simulink model "Discrete_sim_3R_scalar"  (R2024b)
settings: Solver=FixedStepAuto  StartTime=0.0  StopTime=22  FixedStep=0.1  MaxStep=0.1  RelTol=1e-3
libraries: simulink x1
(part 1 of 2)
settings Model: Creator=RSL  LastModifiedBy=cwaight
settings SolverCC: AlgebraicLoopSolver=TrustRegion
settings DataIOCC: ReturnWorkspaceOutputs=off
settings DebuggingCC: UnconnectedInputMsg=warning  UnconnectedOutputMsg=warning  UnconnectedLineMsg=warning  UnderSpecifiedDimensionMsg=warning  ArithmeticOperatorsInVariantConditions=warning
settings ModelReferenceCC: EnableRefExpFcnMdlSchedulingChecks=on
settings SFSimCC: SimUseLocalCustomCode=off  CustomCodeUndefinedFunction=UseInterfaceOnly
settings RTWCC: RTWUseLocalCustomCode=off  GPUComputeCapability=3.5
settings CodeAppCC: StateflowObjectComments=on

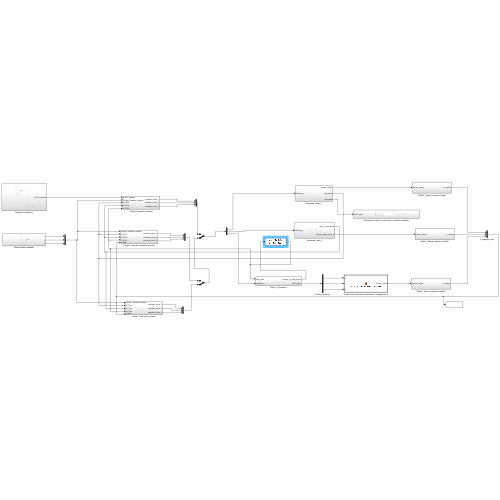
[thumbnail: Simulink's stored preview of the top-level diagram]
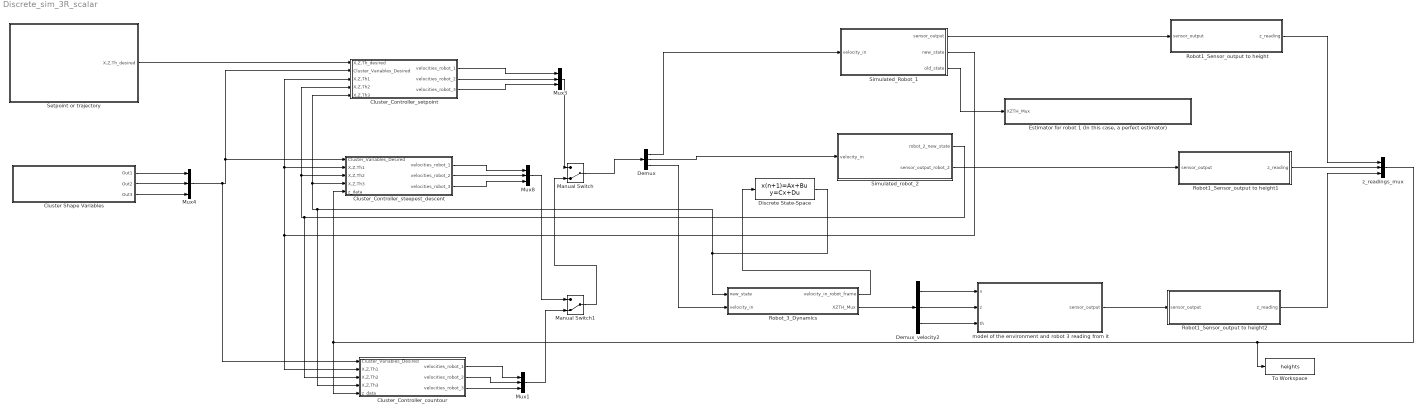
== system Discrete_sim_3R_scalar ==
  Cluster Shape Variables : Subsystem
  Cluster_Controller_countour : Subsystem
  Cluster_Controller_setpoint : Subsystem
  Cluster_Controller_steepest_descent : Subsystem
  Demux : Demux  Outputs=3
  Demux_velocity2 : Demux  Outputs=3
  Discrete State-Space : DiscreteStateSpace  A=[1 0 0; 0 1 0; 0 0 1]  B=[0.1 0 0; 0 0.10 0; 0 0 0.1]  C=[1 0 0; 0 1 0; 0 0 1]  D=[0 0 0; 0 0 0; 0 0 0]  InitialCondition=[-0.85,-1.1,0.1]  SampleTime=-1
  "Estimator for robot 1 (In this case, a perfect estimator)" : Subsystem
  Manual Switch : ManualSwitch  CurrentSetting=0
  Manual Switch1 : ManualSwitch  CurrentSetting=0
  Mux{1,3..4,8} (4 alike) : Mux  Inputs=3
  Robot1_Sensor_output to height : Subsystem
  Robot1_Sensor_output to height1 : Subsystem
  Robot1_Sensor_output to height2 : Subsystem
  Robot_3_Dynamics : Subsystem
  Setpoint or trajectory : Subsystem
  Simulated_Robot_1 : Subsystem
  Simulated_robot_2 : Subsystem
  To Workspace : ToWorkspace  VariableName=heights  SaveFormat=Timeseries  SampleTime=-1
  model of the environment and robot 3 reading from it : MATLAB Function  TreatAsAtomicUnit=on
  z_readings_mux : Mux  Inputs=3
  wires:
  Cluster_Controller_setpoint/1(velocities_robot_1) -> Mux3/1
  Cluster_Controller_setpoint/3(velocities_robot_3) -> Mux3/3
  Cluster_Controller_setpoint/2(velocities_robot_2) -> Mux3/2
  Mux4/1 -> Cluster_Controller_countour/1(Cluster_Variables_Desired), Cluster_Controller_steepest_descent/1(Cluster_Variables_Desired), Cluster_Controller_setpoint/2(Cluster_Variables_Desired)
  Cluster Shape Variables/1(Out1) -> Mux4/1
  Cluster Shape Variables/3(Out3) -> Mux4/3
  Setpoint or trajectory/1(X,Z,Th_desired) -> Cluster_Controller_setpoint/1(X,Z,Th_desired)
  Robot1_Sensor_output to height/1(z_reading) -> z_readings_mux/1
  Cluster_Controller_steepest_descent/3(velocities_robot_3) -> Mux8/3
  Cluster_Controller_steepest_descent/2(velocities_robot_2) -> Mux8/2
  Cluster_Controller_steepest_descent/1(velocities_robot_1) -> Mux8/1
  Cluster Shape Variables/2(Out2) -> Mux4/2
  Demux_velocity2/1 -> model of the environment and robot 3 reading from it/1(x)
  model of the environment and robot 3 reading from it/1(sensor_output) -> Robot1_Sensor_output to height2/1(sensor_output)
  Demux_velocity2/2 -> model of the environment and robot 3 reading from it/2(z)
  Demux_velocity2/3 -> model of the environment and robot 3 reading from it/3(th)
  Robot1_Sensor_output to height1/1(z_reading) -> z_readings_mux/2
  Robot1_Sensor_output to height2/1(z_reading) -> z_readings_mux/3
  Robot_3_Dynamics/2(XZTH_Mux) -> Demux_velocity2/1
  z_readings_mux/1 -> Cluster_Controller_steepest_descent/5(z_data), Cluster_Controller_countour/5(z_data), To Workspace/1
  Robot_3_Dynamics/1(velocity_in_robot_frame) -> Discrete State-Space/1
  Discrete State-Space/1 -> Robot_3_Dynamics/1(new_state), Cluster_Controller_countour/4(X,Z,Th3), Cluster_Controller_steepest_descent/4(X,Z,Th3), Cluster_Controller_setpoint/5(X,Z,Th3)
  Mux3/1 -> Manual Switch/1
  Simulated_Robot_1/2(new_state) -> Cluster_Controller_setpoint/3(X,Z,Th1), Cluster_Controller_steepest_descent/2(X,Z,Th1), Cluster_Controller_countour/2(X,Z,Th1)
  Simulated_Robot_1/1(sensor_output) -> Robot1_Sensor_output to height/1(sensor_output)
  Simulated_Robot_1/3(old_state) -> "Estimator for robot 1 (In this case, a perfect estimator)"/1(XZTH_Mux)
  Demux/1 -> Simulated_Robot_1/1(velocity_in)
  Manual Switch/1 -> Demux/1
  Simulated_robot_2/1(robot_2_new_state) -> Cluster_Controller_countour/3(X,Z,Th2), Cluster_Controller_setpoint/4(X,Z,Th2), Cluster_Controller_steepest_descent/3(X,Z,Th2)
  Demux/2 -> Simulated_robot_2/1(velocity_in)
  Simulated_robot_2/2(sensor_output_robot_2) -> Robot1_Sensor_output to height1/1(sensor_output)
  Demux/3 -> Robot_3_Dynamics/2(velocity_in)
  Manual Switch1/1 -> Manual Switch/2
  Mux8/1 -> Manual Switch1/1
  Mux1/1 -> Manual Switch1/2
  Cluster_Controller_countour/1(velocities_robot_1) -> Mux1/1
  Cluster_Controller_countour/2(velocities_robot_2) -> Mux1/2
  Cluster_Controller_countour/3(velocities_robot_3) -> Mux1/3

== system Discrete_sim_3R_scalar/Cluster Shape Variables ==
  Cluster Variable C : Constant  Value=pi/2
  Cluster_Variable_B : Constant  Value=0.35
  Cluster_variable_A : Constant  Value=0.35
  Out1 : Outport
  Out2 : Outport  Port=2
  Out3 : Outport  Port=3
  wires:
  Cluster_variable_A/1 -> Out1/1
  Cluster Variable C/1 -> Out3/1
  Cluster_Variable_B/1 -> Out2/1

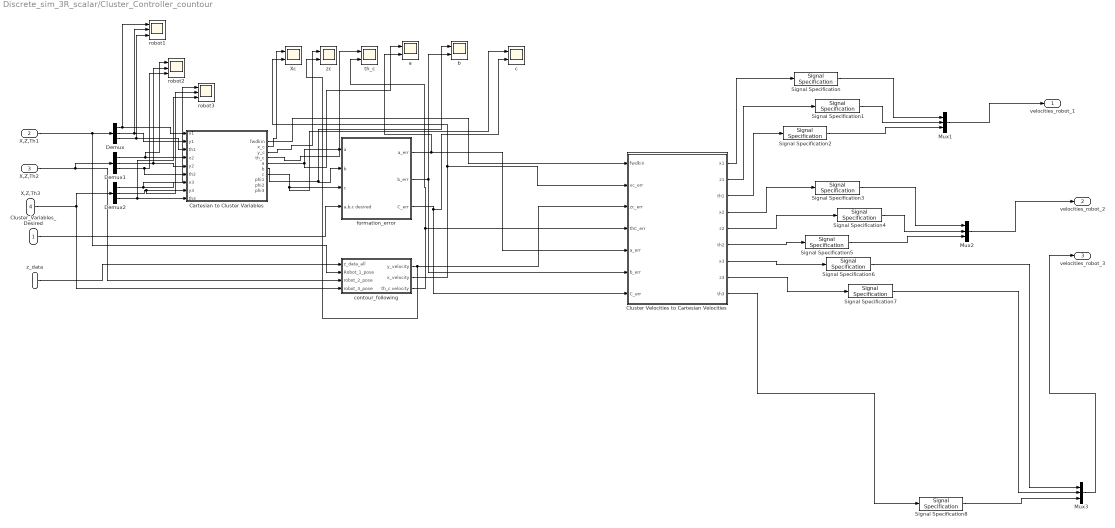
== system Discrete_sim_3R_scalar/Cluster_Controller_countour ==
  Cluster_Variables_Desired : Inport
  X,Z,Th1 : Inport  Port=2
  X,Z,Th2 : Inport  Port=3
  X,Z,Th3 : Inport  Port=4
  z_data : Inport  Port=5
  Cartesian to Cluster Variables : MATLAB Function  TreatAsAtomicUnit=on
  Cluster Velocities to Cartesian Velocities : MATLAB Function  TreatAsAtomicUnit=on
  Demux : Demux  Outputs=3
  Demux1 : Demux  Outputs=3
  Demux2 : Demux  Outputs=3
  Mux1 : Mux  Inputs=3
  Mux2 : Mux  Inputs=3
  Mux3 : Mux  Inputs=3
  Signal Specification{,1..8} (9 alike) : SignalSpecification  Dimensions=1
  Xc : Scope  NumInputPorts=2
  a : Scope  NumInputPorts=2
  b : Scope  NumInputPorts=2
  c : Scope  NumInputPorts=2
  contour_following : Subsystem
  formation_error : Subsystem
  robot1 : Scope  NumInputPorts=3
  robot2 : Scope  NumInputPorts=3
  robot3 : Scope  NumInputPorts=3
  th_c : Scope  NumInputPorts=2
  zc : Scope  NumInputPorts=2
  velocities_robot_1 : Outport
  velocities_robot_2 : Outport  Port=2
  velocities_robot_3 : Outport  Port=3
  wires:
  X,Z,Th1/1 -> contour_following/2(Robot_1_pose), Demux/1
  X,Z,Th2/1 -> contour_following/3(robot_2_pose), Demux1/1
  X,Z,Th3/1 -> Demux2/1, contour_following/4(robot_3_pose)
  Demux/1 -> robot1/1, Cartesian to Cluster Variables/1(x1)
  Demux/2 -> robot1/2, Cartesian to Cluster Variables/2(y1)
  Demux/3 -> robot1/3, Cartesian to Cluster Variables/3(th1)
  Demux1/1 -> robot2/1, Cartesian to Cluster Variables/4(x2)
  Demux1/2 -> robot2/2, Cartesian to Cluster Variables/5(y2)
  Demux1/3 -> robot2/3, Cartesian to Cluster Variables/6(th2)
  Demux2/1 -> robot3/1, Cartesian to Cluster Variables/7(x3)
  Demux2/2 -> robot3/2, Cartesian to Cluster Variables/8(y3)
  Demux2/3 -> robot3/3, Cartesian to Cluster Variables/9(th3)
  Cartesian to Cluster Variables/2(x_c) -> Xc/1
  Cartesian to Cluster Variables/3(y_c) -> zc/1
  Cartesian to Cluster Variables/4(th_c) -> th_c/1
  Cartesian to Cluster Variables/5(a) -> a/1, formation_error/1(a)
  Cartesian to Cluster Variables/6(b) -> formation_error/2(b), b/1
  Cartesian to Cluster Variables/7(c) -> c/1, formation_error/3(c)
  Cluster_Variables_Desired/1 -> formation_error/4(a,b,c desired)
  formation_error/1(a_err) -> Cluster Velocities to Cartesian Velocities/5(a_err), a/2
  formation_error/2(b_err) -> Cluster Velocities to Cartesian Velocities/6(b_err), b/2
  formation_error/3(C_err) -> Cluster Velocities to Cartesian Velocities/7(C_err), c/2
  Cartesian to Cluster Variables/1(fwdkin) -> Cluster Velocities to Cartesian Velocities/1(fwdkin)
  z_data/1 -> contour_following/1(z_data_all)
  contour_following/2(x_velocity) -> Cluster Velocities to Cartesian Velocities/2(xc_err), Xc/2
  contour_following/1(y_velocity) -> Cluster Velocities to Cartesian Velocities/3(zc_err), zc/2
  contour_following/3(th_c velocity) -> th_c/2, Cluster Velocities to Cartesian Velocities/4(thC_err)
  Signal Specification/1 -> Mux1/1
  Cluster Velocities to Cartesian Velocities/1(x1) -> Signal Specification/1
  Cluster Velocities to Cartesian Velocities/5(z2) -> Signal Specification4/1
  Signal Specification7/1 -> Mux3/2
  Cluster Velocities to Cartesian Velocities/7(x3) -> Signal Specification6/1
  Cluster Velocities to Cartesian Velocities/6(th2) -> Signal Specification5/1
  Mux1/1 -> velocities_robot_1/1
  Cluster Velocities to Cartesian Velocities/4(x2) -> Signal Specification3/1
  Signal Specification1/1 -> Mux1/2
  Signal Specification8/1 -> Mux3/3
  Signal Specification6/1 -> Mux3/1
  Signal Specification3/1 -> Mux2/1
  Signal Specification5/1 -> Mux2/3
  Signal Specification2/1 -> Mux1/3
  Cluster Velocities to Cartesian Velocities/3(th1) -> Signal Specification2/1
  Mux3/1 -> velocities_robot_3/1
  Signal Specification4/1 -> Mux2/2
  Cluster Velocities to Cartesian Velocities/9(th3) -> Signal Specification8/1
  Cluster Velocities to Cartesian Velocities/2(z1) -> Signal Specification1/1
  Mux2/1 -> velocities_robot_2/1
  Cluster Velocities to Cartesian Velocities/8(z3) -> Signal Specification7/1

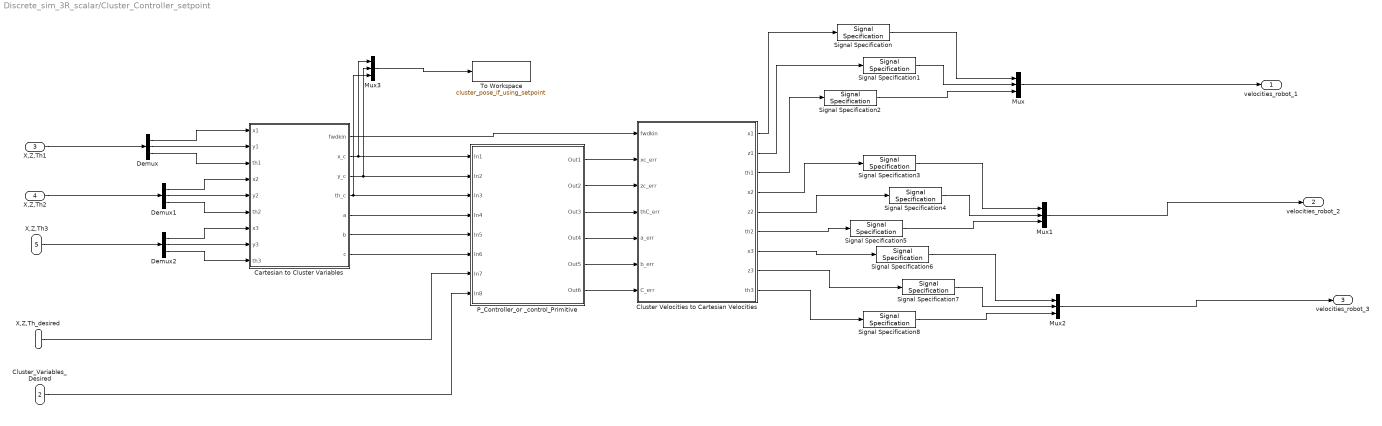
== system Discrete_sim_3R_scalar/Cluster_Controller_setpoint ==
  X,Z,Th_desired : Inport
  Cluster_Variables_Desired : Inport  Port=2
  X,Z,Th1 : Inport  Port=3
  X,Z,Th2 : Inport  Port=4
  X,Z,Th3 : Inport  Port=5
  Cartesian to Cluster Variables : MATLAB Function  TreatAsAtomicUnit=on
  Cluster Velocities to Cartesian Velocities : MATLAB Function  TreatAsAtomicUnit=on
  Demux : Demux  Outputs=3
  Demux1 : Demux  Outputs=3
  Demux2 : Demux  Outputs=3
  Mux{,1..3} (4 alike) : Mux  Inputs=3
  P_Controller_or _control_Primitive : Subsystem
  Signal Specification{,1..8} (9 alike) : SignalSpecification  Dimensions=1
  To Workspace : ToWorkspace  VariableName=cluster_pose_if_using_setpoint  SampleTime=-1
  velocities_robot_1 : Outport
  velocities_robot_2 : Outport  Port=2
  velocities_robot_3 : Outport  Port=3
  wires:
  X,Z,Th1/1 -> Demux/1
  X,Z,Th2/1 -> Demux1/1
  X,Z,Th3/1 -> Demux2/1
  Demux/1 -> Cartesian to Cluster Variables/1(x1)
  Demux/2 -> Cartesian to Cluster Variables/2(y1)
  Demux/3 -> Cartesian to Cluster Variables/3(th1)
  Demux1/1 -> Cartesian to Cluster Variables/4(x2)
  Demux1/2 -> Cartesian to Cluster Variables/5(y2)
  Demux1/3 -> Cartesian to Cluster Variables/6(th2)
  Demux2/1 -> Cartesian to Cluster Variables/7(x3)
  Demux2/2 -> Cartesian to Cluster Variables/8(y3)
  Demux2/3 -> Cartesian to Cluster Variables/9(th3)
  Cartesian to Cluster Variables/2(x_c) -> Mux3/1, P_Controller_or _control_Primitive/1(In1)
  Cartesian to Cluster Variables/3(y_c) -> Mux3/2, P_Controller_or _control_Primitive/2(In2)
  Cartesian to Cluster Variables/4(th_c) -> P_Controller_or _control_Primitive/3(In3), Mux3/3
  Cartesian to Cluster Variables/5(a) -> P_Controller_or _control_Primitive/4(In4)
  Cartesian to Cluster Variables/6(b) -> P_Controller_or _control_Primitive/5(In5)
  Cartesian to Cluster Variables/7(c) -> P_Controller_or _control_Primitive/6(In6)
  X,Z,Th_desired/1 -> P_Controller_or _control_Primitive/7(In7)
  Cluster_Variables_Desired/1 -> P_Controller_or _control_Primitive/8(In8)
  P_Controller_or _control_Primitive/1(Out1) -> Cluster Velocities to Cartesian Velocities/2(xc_err)
  P_Controller_or _control_Primitive/2(Out2) -> Cluster Velocities to Cartesian Velocities/3(zc_err)
  P_Controller_or _control_Primitive/3(Out3) -> Cluster Velocities to Cartesian Velocities/4(thC_err)
  P_Controller_or _control_Primitive/4(Out4) -> Cluster Velocities to Cartesian Velocities/5(a_err)
  P_Controller_or _control_Primitive/5(Out5) -> Cluster Velocities to Cartesian Velocities/6(b_err)
  P_Controller_or _control_Primitive/6(Out6) -> Cluster Velocities to Cartesian Velocities/7(C_err)
  Cartesian to Cluster Variables/1(fwdkin) -> Cluster Velocities to Cartesian Velocities/1(fwdkin)
  Mux/1 -> velocities_robot_1/1
  Signal Specification/1 -> Mux/1
  Cluster Velocities to Cartesian Velocities/1(x1) -> Signal Specification/1
  Signal Specification1/1 -> Mux/2
  Cluster Velocities to Cartesian Velocities/2(z1) -> Signal Specification1/1
  Signal Specification2/1 -> Mux/3
  Cluster Velocities to Cartesian Velocities/3(th1) -> Signal Specification2/1
  Signal Specification3/1 -> Mux1/1
  Cluster Velocities to Cartesian Velocities/4(x2) -> Signal Specification3/1
  Mux1/1 -> velocities_robot_2/1
  Signal Specification4/1 -> Mux1/2
  Signal Specification5/1 -> Mux1/3
  Cluster Velocities to Cartesian Velocities/6(th2) -> Signal Specification5/1
  Cluster Velocities to Cartesian Velocities/5(z2) -> Signal Specification4/1
  Signal Specification6/1 -> Mux2/1
  Cluster Velocities to Cartesian Velocities/7(x3) -> Signal Specification6/1
  Mux2/1 -> velocities_robot_3/1
  Signal Specification7/1 -> Mux2/2
  Signal Specification8/1 -> Mux2/3
  Cluster Velocities to Cartesian Velocities/9(th3) -> Signal Specification8/1
  Cluster Velocities to Cartesian Velocities/8(z3) -> Signal Specification7/1
  Mux3/1 -> To Workspace/1

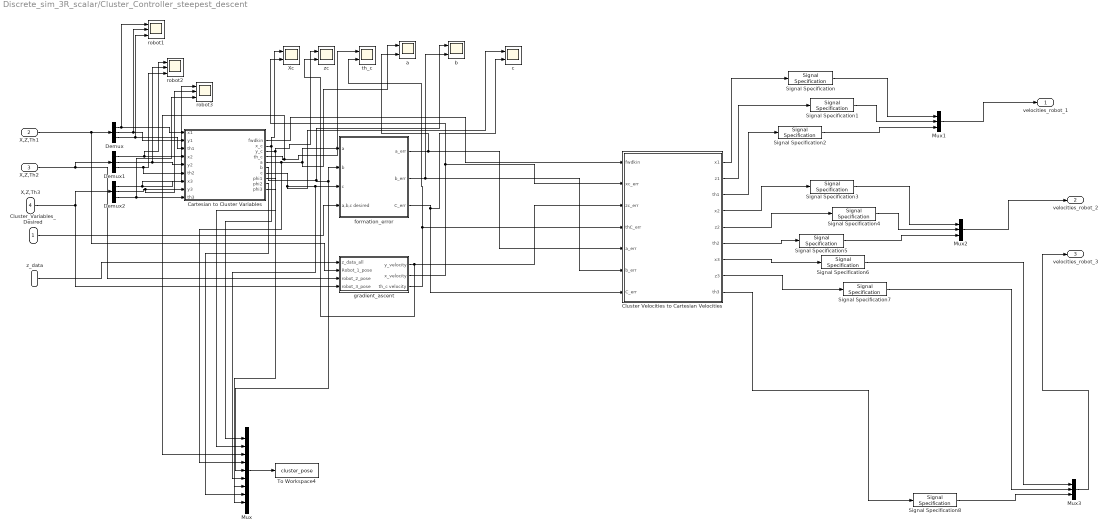
== system Discrete_sim_3R_scalar/Cluster_Controller_steepest_descent ==
  Cluster_Variables_Desired : Inport
  X,Z,Th1 : Inport  Port=2
  X,Z,Th2 : Inport  Port=3
  X,Z,Th3 : Inport  Port=4
  z_data : Inport  Port=5
  Cartesian to Cluster Variables : MATLAB Function  TreatAsAtomicUnit=on
  Cluster Velocities to Cartesian Velocities : MATLAB Function  TreatAsAtomicUnit=on
  Demux : Demux  Outputs=3
  Demux1 : Demux  Outputs=3
  Demux2 : Demux  Outputs=3
  Mux : Mux  Inputs=9
  Mux1 : Mux  Inputs=3
  Mux2 : Mux  Inputs=3
  Mux3 : Mux  Inputs=3
  Signal Specification{,1..8} (9 alike) : SignalSpecification  Dimensions=1
  To Workspace4 : ToWorkspace  VariableName=cluster_pose  SampleTime=-1
  Xc : Scope  NumInputPorts=2
  a : Scope  NumInputPorts=2
  b : Scope  NumInputPorts=2
  c : Scope  NumInputPorts=2
  formation_error : Subsystem
  gradient_ascent : Subsystem
  robot1 : Scope  NumInputPorts=3
  robot2 : Scope  NumInputPorts=3
  robot3 : Scope  NumInputPorts=3
  th_c : Scope  NumInputPorts=2
  zc : Scope  NumInputPorts=2
  velocities_robot_1 : Outport
  velocities_robot_2 : Outport  Port=2
  velocities_robot_3 : Outport  Port=3
  wires:
  X,Z,Th1/1 -> gradient_ascent/2(Robot_1_pose), Demux/1
  X,Z,Th2/1 -> gradient_ascent/3(robot_2_pose), Demux1/1
  X,Z,Th3/1 -> Demux2/1, gradient_ascent/4(robot_3_pose)
  Demux/1 -> robot1/1, Cartesian to Cluster Variables/1(x1)
  Demux/2 -> robot1/2, Cartesian to Cluster Variables/2(y1)
  Demux/3 -> robot1/3, Cartesian to Cluster Variables/3(th1)
  Demux1/1 -> robot2/1, Cartesian to Cluster Variables/4(x2)
  Demux1/2 -> robot2/2, Cartesian to Cluster Variables/5(y2)
  Demux1/3 -> robot2/3, Cartesian to Cluster Variables/6(th2)
  Demux2/1 -> robot3/1, Cartesian to Cluster Variables/7(x3)
  Demux2/2 -> robot3/2, Cartesian to Cluster Variables/8(y3)
  Demux2/3 -> robot3/3, Cartesian to Cluster Variables/9(th3)
  Cartesian to Cluster Variables/2(x_c) -> Xc/1, Mux/1
  Cartesian to Cluster Variables/3(y_c) -> zc/1, Mux/2
  Cartesian to Cluster Variables/4(th_c) -> Mux/3, th_c/1
  Cartesian to Cluster Variables/5(a) -> a/1, formation_error/1(a), Mux/4
  Cartesian to Cluster Variables/6(b) -> formation_error/2(b), Mux/5, b/1
  Cartesian to Cluster Variables/7(c) -> c/1, Mux/6, formation_error/3(c)
  Cluster_Variables_Desired/1 -> formation_error/4(a,b,c desired)
  formation_error/1(a_err) -> Cluster Velocities to Cartesian Velocities/5(a_err), a/2
  formation_error/2(b_err) -> Cluster Velocities to Cartesian Velocities/6(b_err), b/2
  formation_error/3(C_err) -> Cluster Velocities to Cartesian Velocities/7(C_err), c/2
  Cartesian to Cluster Variables/1(fwdkin) -> Cluster Velocities to Cartesian Velocities/1(fwdkin)
  z_data/1 -> gradient_ascent/1(z_data_all)
  gradient_ascent/2(x_velocity) -> Cluster Velocities to Cartesian Velocities/2(xc_err), Xc/2
  gradient_ascent/1(y_velocity) -> Cluster Velocities to Cartesian Velocities/3(zc_err), zc/2
  gradient_ascent/3(th_c velocity) -> th_c/2, Cluster Velocities to Cartesian Velocities/4(thC_err)
  Mux/1 -> To Workspace4/1
  Cartesian to Cluster Variables/8(phi1) -> Mux/7
  Cartesian to Cluster Variables/9(phi2) -> Mux/8
  Cartesian to Cluster Variables/10(phi3) -> Mux/9
  Signal Specification/1 -> Mux1/1
  Cluster Velocities to Cartesian Velocities/1(x1) -> Signal Specification/1
  Cluster Velocities to Cartesian Velocities/5(z2) -> Signal Specification4/1
  Signal Specification7/1 -> Mux3/2
  Cluster Velocities to Cartesian Velocities/7(x3) -> Signal Specification6/1
  Cluster Velocities to Cartesian Velocities/6(th2) -> Signal Specification5/1
  Mux1/1 -> velocities_robot_1/1
  Cluster Velocities to Cartesian Velocities/4(x2) -> Signal Specification3/1
  Signal Specification1/1 -> Mux1/2
  Signal Specification8/1 -> Mux3/3
  Signal Specification6/1 -> Mux3/1
  Signal Specification3/1 -> Mux2/1
  Signal Specification5/1 -> Mux2/3
  Signal Specification2/1 -> Mux1/3
  Cluster Velocities to Cartesian Velocities/3(th1) -> Signal Specification2/1
  Mux3/1 -> velocities_robot_3/1
  Signal Specification4/1 -> Mux2/2
  Cluster Velocities to Cartesian Velocities/9(th3) -> Signal Specification8/1
  Cluster Velocities to Cartesian Velocities/2(z1) -> Signal Specification1/1
  Mux2/1 -> velocities_robot_2/1
  Cluster Velocities to Cartesian Velocities/8(z3) -> Signal Specification7/1

== system Discrete_sim_3R_scalar/Estimator for robot 1 (In this case, a perfect estimator) ==
  XZTH_Mux : Inport
  Demux_velocity2 : Demux  Outputs=3
  Same Crater Yet Again : MATLAB Function  TreatAsAtomicUnit=on
  To Workspace6 : ToWorkspace  VariableName=sensor1_estimate  SampleTime=-1
  wires:
  Same Crater Yet Again/1(sensor_output) -> To Workspace6/1
  Demux_velocity2/3 -> Same Crater Yet Again/3(th)
  XZTH_Mux/1 -> Demux_velocity2/1
  Demux_velocity2/2 -> Same Crater Yet Again/2(z)
  Demux_velocity2/1 -> Same Crater Yet Again/1(x)

== system Discrete_sim_3R_scalar/Robot1_Sensor_output to height ==
  sensor_output : Inport
  Mountain : MATLAB Function  TreatAsAtomicUnit=on
  z_reading : Outport
  wires:
  sensor_output/1 -> Mountain/1(sensor_output)
  Mountain/1(height) -> z_reading/1

== system Discrete_sim_3R_scalar/Robot1_Sensor_output to height1 ==
  sensor_output : Inport
  Mountain : MATLAB Function  TreatAsAtomicUnit=on
  z_reading : Outport
  wires:
  sensor_output/1 -> Mountain/1(sensor_output)
  Mountain/1(height) -> z_reading/1

== system Discrete_sim_3R_scalar/Robot1_Sensor_output to height2 ==
  sensor_output : Inport
  Mountain : MATLAB Function  TreatAsAtomicUnit=on
  z_reading : Outport
  wires:
  sensor_output/1 -> Mountain/1(sensor_output)
  Mountain/1(height) -> z_reading/1

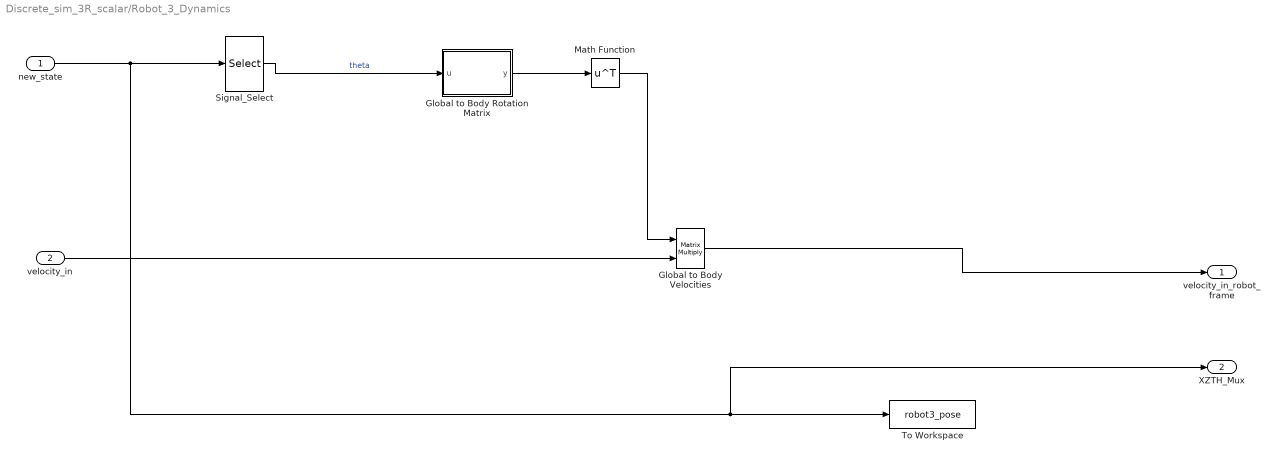
== system Discrete_sim_3R_scalar/Robot_3_Dynamics ==
  new_state : Inport
  velocity_in : Inport  Port=2
  Global to Body Velocities : Product  Multiplication=Matrix(*)
  Global to Body Rotation Matrix : MATLAB Function  TreatAsAtomicUnit=on
  Math Function : Math  Operator=transpose  SignedPower=on
  Signal_Select : Selector  InputPortWidth=3  IndexOptions=Index vector (dialog)  Indices=[3]  OutputSizes=1
  To Workspace : ToWorkspace  VariableName=robot3_pose  SaveFormat=Timeseries  SampleTime=-1
  velocity_in_robot_frame : Outport
  XZTH_Mux : Outport  Port=2
  wires:
  Signal_Select/1 -> Global to Body Rotation Matrix/1(u)  "theta"
  Global to Body Velocities/1 -> velocity_in_robot_frame/1
  new_state/1 -> XZTH_Mux/1, To Workspace/1, Signal_Select/1
  velocity_in/1 -> Global to Body Velocities/2
  Global to Body Rotation Matrix/1(y) -> Math Function/1
  Math Function/1 -> Global to Body Velocities/1

== system Discrete_sim_3R_scalar/Setpoint or trajectory ==
  Manual Switch : ManualSwitch
  Mux3 : Mux  Inputs=3
  Ramp : simulink/Sources/Ramp  slope=1  start=0  InitialOutput=0.1
  "Theta_Set Point1 " : Constant  Value=0.1
  X_Set Point : Constant  Value=1.5
  Z_Set Point1 : Constant  Value=0.5
  X,Z,Th_desired : Outport
  wires:
  Mux3/1 -> X,Z,Th_desired/1
  Z_Set Point1/1 -> Mux3/2
  Manual Switch/1 -> Mux3/3
  "Theta_Set Point1 "/1 -> Manual Switch/1
  X_Set Point/1 -> Mux3/1
  Ramp/1 -> Manual Switch/2

== system Discrete_sim_3R_scalar/Simulated_Robot_1 ==
  velocity_in : Inport
  Crater : MATLAB Function  TreatAsAtomicUnit=on
  Demux_velocity : Demux  Outputs=3
  Discrete State-Space : DiscreteStateSpace  A=[1 0 0; 0 1 0; 0 0 1]  B=[0.1 0 0; 0 0.10 0; 0 0 0.1]  C=[1 0 0; 0 1 0; 0 0 1]  D=[0 0 0; 0 0 0; 0 0 0]  InitialCondition=[-1,-1,0]  SampleTime=-1
  Robot_signal_processing_1 : Subsystem
  sensor_output : Outport
  new_state : Outport  Port=2
  old_state : Outport  Port=3
  wires:
  Crater/1(sensor_output) -> sensor_output/1
  Demux_velocity/1 -> Crater/1(x)
  Demux_velocity/3 -> Crater/3(th)
  Robot_signal_processing_1/2(XZTH_Mux) -> old_state/1, Demux_velocity/1
  velocity_in/1 -> Robot_signal_processing_1/2(velocity_in)
  Discrete State-Space/1 -> Robot_signal_processing_1/1(robot_1_pose), new_state/1
  Demux_velocity/2 -> Crater/2(z)
  Robot_signal_processing_1/1(velocity_in_robot_frame) -> Discrete State-Space/1

== system Discrete_sim_3R_scalar/Simulated_robot_2 ==
  velocity_in : Inport
  Demux_velocity1 : Demux  Outputs=3
  Discrete State-Space : DiscreteStateSpace  A=[1 0 0; 0 1 0; 0 0 1]  B=[0.1 0 0; 0 0.10 0; 0 0 0.1]  C=[1 0 0; 0 1 0; 0 0 1]  D=[0 0 0; 0 0 0; 0 0 0]  InitialCondition=[-1.1,-1.1,0]  SampleTime=-1
  Robot_signal_processing_2 : Subsystem
  Same Crater : MATLAB Function  TreatAsAtomicUnit=on
  robot_2_new_state : Outport
  sensor_output_robot_2 : Outport  Port=2
  wires:
  Demux_velocity1/1 -> Same Crater/1(x)
  Demux_velocity1/3 -> Same Crater/3(th)
  Same Crater/1(sensor_output) -> sensor_output_robot_2/1
  Demux_velocity1/2 -> Same Crater/2(z)
  velocity_in/1 -> Robot_signal_processing_2/2(velocity_in)
  Discrete State-Space/1 -> robot_2_new_state/1, Robot_signal_processing_2/1(robot_2)
  Robot_signal_processing_2/2(XZTH_Mux) -> Demux_velocity1/1
  Robot_signal_processing_2/1(velocity_in_robot_frame) -> Discrete State-Space/1

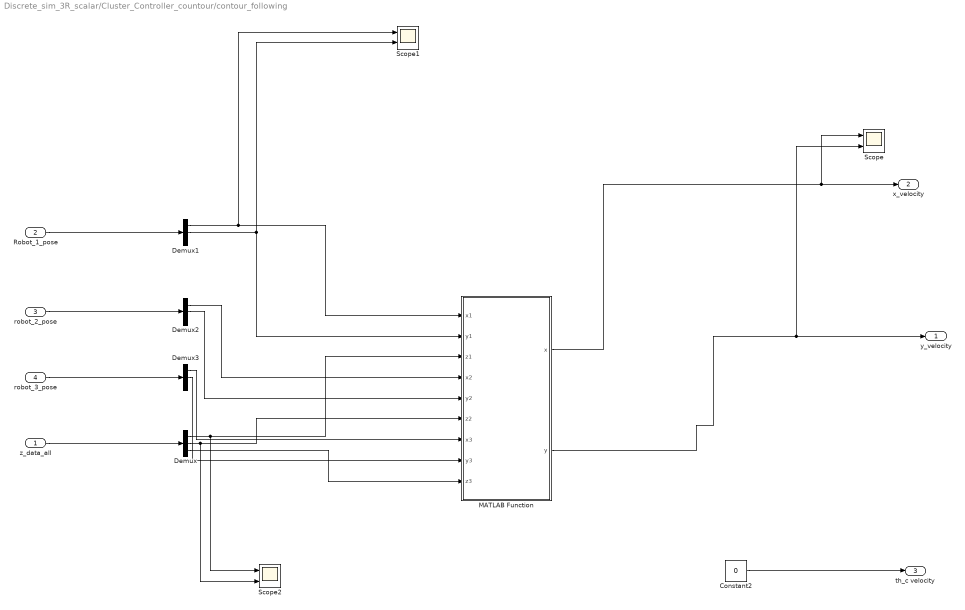
== system Discrete_sim_3R_scalar/Cluster_Controller_countour/contour_following ==
  z_data_all : Inport
  Robot_1_pose : Inport  Port=2
  robot_2_pose : Inport  Port=3
  robot_3_pose : Inport  Port=4
  Constant2 : Constant  Value=0
  Demux{,1..3} (4 alike) : Demux  Outputs=3
  MATLAB Function : MATLAB Function  TreatAsAtomicUnit=on
  Scope : Scope  NumInputPorts=2
  Scope1 : Scope  NumInputPorts=2
  Scope2 : Scope  NumInputPorts=2
  y_velocity : Outport
  x_velocity : Outport  Port=2
  th_c velocity : Outport  Port=3
  wires:
  Constant2/1 -> th_c velocity/1
  z_data_all/1 -> Demux/1
  Robot_1_pose/1 -> Demux1/1
  robot_2_pose/1 -> Demux2/1
  robot_3_pose/1 -> Demux3/1
  Demux1/1 -> Scope1/1, MATLAB Function/1(x1)
  Demux1/2 -> MATLAB Function/2(y1), Scope1/2
  Demux/1 -> Scope2/1, MATLAB Function/3(z1)
  Demux2/1 -> MATLAB Function/4(x2)
  Demux2/2 -> MATLAB Function/5(y2)
  Demux/2 -> Scope2/2, MATLAB Function/6(z2)
  Demux3/1 -> MATLAB Function/7(x3)
  Demux3/2 -> MATLAB Function/8(y3)
  Demux/3 -> MATLAB Function/9(z3)
  MATLAB Function/1(x) -> Scope/1, x_velocity/1
  MATLAB Function/2(y) -> Scope/2, y_velocity/1

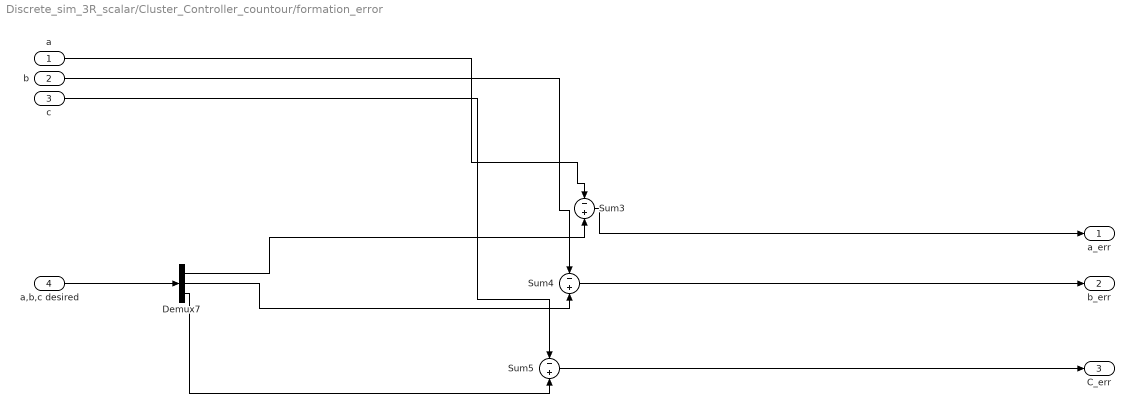
== system Discrete_sim_3R_scalar/Cluster_Controller_countour/formation_error ==
  a : Inport
  b : Inport  Port=2
  c : Inport  Port=3
  a,b,c desired : Inport  Port=4
  Demux7 : Demux  Outputs=3
  Sum3 : Sum  Inputs=-+
  Sum4 : Sum  Inputs=-+
  Sum5 : Sum  Inputs=-+
  a_err : Outport
  b_err : Outport  Port=2
  C_err : Outport  Port=3
  wires:
  Sum3/1 -> a_err/1
  Demux7/3 -> Sum5/2
  a,b,c desired/1 -> Demux7/1
  Demux7/1 -> Sum3/2
  b/1 -> Sum4/1
  Demux7/2 -> Sum4/2
  c/1 -> Sum5/1
  Sum4/1 -> b_err/1
  Sum5/1 -> C_err/1
  a/1 -> Sum3/1

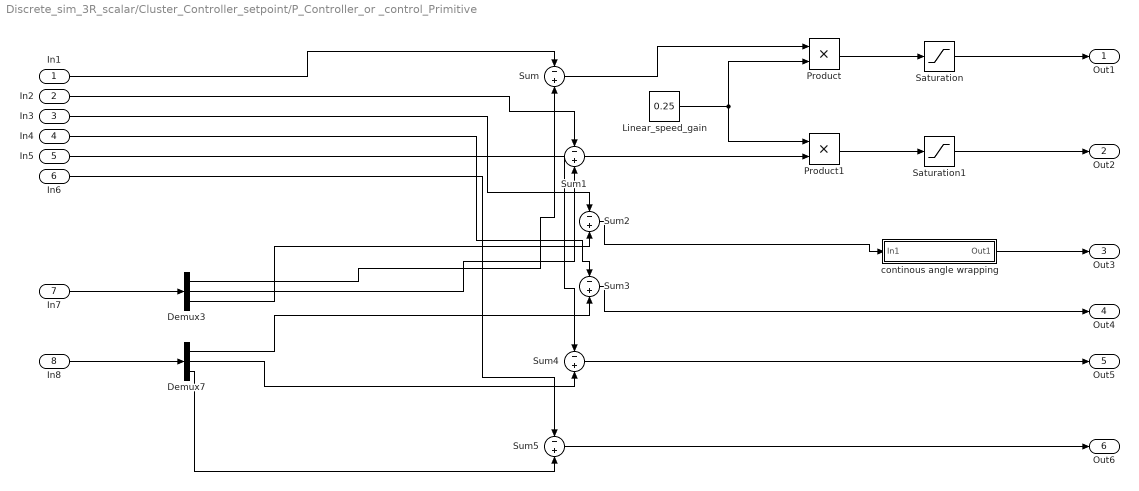
== system Discrete_sim_3R_scalar/Cluster_Controller_setpoint/P_Controller_or _control_Primitive ==
  In1 : Inport
  In2 : Inport  Port=2
  In3 : Inport  Port=3
  In4 : Inport  Port=4
  In5 : Inport  Port=5
  In6 : Inport  Port=6
  In7 : Inport  Port=7
  In8 : Inport  Port=8
  Demux3 : Demux  Outputs=3
  Demux7 : Demux  Outputs=3
  Linear_speed_gain : Constant  Value=0.25
  Product : Product
  Product1 : Product
  Saturation : Saturate
  Saturation1 : Saturate
  Sum{,1..5} (6 alike) : Sum  Inputs=-+
  continous angle wrapping : Subsystem
  Out1 : Outport
  Out2 : Outport  Port=2
  Out3 : Outport  Port=3
  Out4 : Outport  Port=4
  Out5 : Outport  Port=5
  Out6 : Outport  Port=6
  wires:
  In3/1 -> Sum2/1
  Demux3/2 -> Sum1/2
  Sum3/1 -> Out4/1
  In2/1 -> Sum1/1
  Demux3/3 -> Sum2/2
  Demux7/3 -> Sum5/2
  In8/1 -> Demux7/1
  Demux7/1 -> Sum3/2
  In1/1 -> Sum/1
  In5/1 -> Sum4/1
  Demux7/2 -> Sum4/2
  In6/1 -> Sum5/1
  Sum4/1 -> Out5/1
  Sum5/1 -> Out6/1
  Demux3/1 -> Sum/2
  In4/1 -> Sum3/1
  In7/1 -> Demux3/1
  Sum2/1 -> continous angle wrapping/1(In1)
  continous angle wrapping/1(Out1) -> Out3/1
  Sum/1 -> Product/1
  Linear_speed_gain/1 -> Product/2, Product1/1
  Sum1/1 -> Product1/2
  Saturation/1 -> Out1/1
  Product/1 -> Saturation/1
  Product1/1 -> Saturation1/1
  Saturation1/1 -> Out2/1

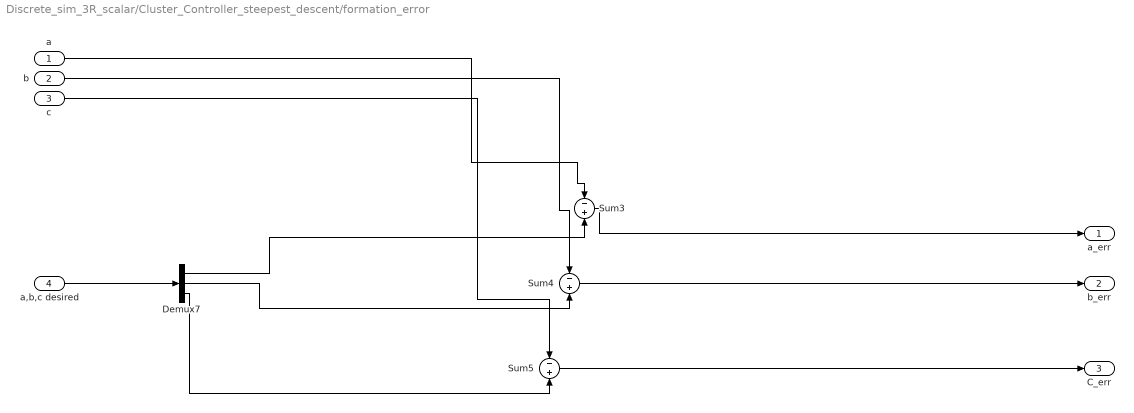
== system Discrete_sim_3R_scalar/Cluster_Controller_steepest_descent/formation_error ==
  a : Inport
  b : Inport  Port=2
  c : Inport  Port=3
  a,b,c desired : Inport  Port=4
  Demux7 : Demux  Outputs=3
  Sum3 : Sum  Inputs=-+
  Sum4 : Sum  Inputs=-+
  Sum5 : Sum  Inputs=-+
  a_err : Outport
  b_err : Outport  Port=2
  C_err : Outport  Port=3
  wires:
  Sum3/1 -> a_err/1
  Demux7/3 -> Sum5/2
  a,b,c desired/1 -> Demux7/1
  Demux7/1 -> Sum3/2
  b/1 -> Sum4/1
  Demux7/2 -> Sum4/2
  c/1 -> Sum5/1
  Sum4/1 -> b_err/1
  Sum5/1 -> C_err/1
  a/1 -> Sum3/1

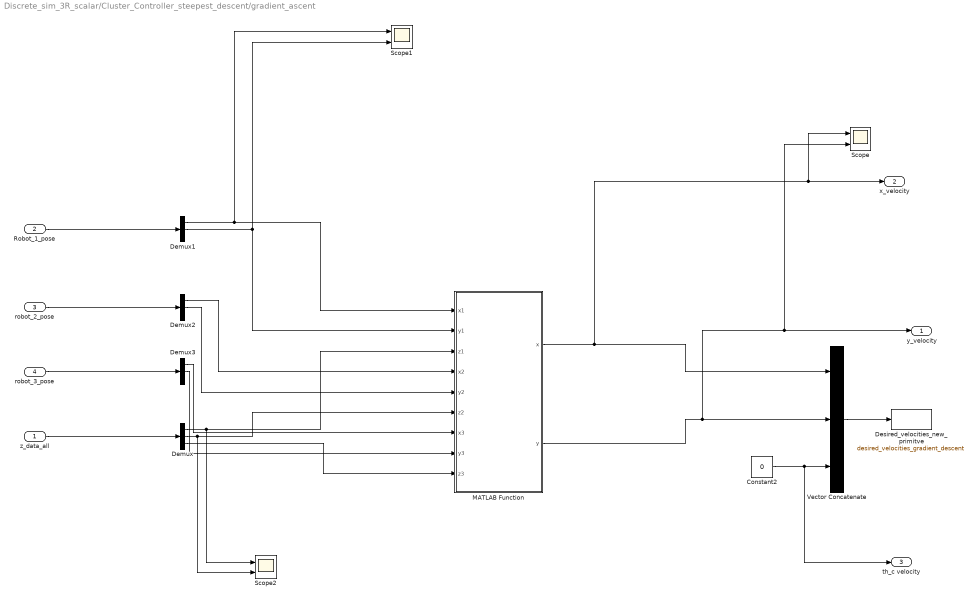
== system Discrete_sim_3R_scalar/Cluster_Controller_steepest_descent/gradient_ascent ==
  z_data_all : Inport
  Robot_1_pose : Inport  Port=2
  robot_2_pose : Inport  Port=3
  robot_3_pose : Inport  Port=4
  Constant2 : Constant  Value=0
  Demux{,1..3} (4 alike) : Demux  Outputs=3
  Desired_velocities_new_primitve : ToWorkspace  VariableName=desired_velocities_gradient_descent  SampleTime=-1
  MATLAB Function : MATLAB Function  TreatAsAtomicUnit=on
  Scope : Scope  NumInputPorts=2
  Scope1 : Scope  NumInputPorts=2
  Scope2 : Scope  NumInputPorts=2
  Vector Concatenate : Concatenate  NumInputs=3
  y_velocity : Outport
  x_velocity : Outport  Port=2
  th_c velocity : Outport  Port=3
  wires:
  Vector Concatenate/1 -> Desired_velocities_new_primitve/1
  Constant2/1 -> th_c velocity/1, Vector Concatenate/3
  z_data_all/1 -> Demux/1
  Robot_1_pose/1 -> Demux1/1
  robot_2_pose/1 -> Demux2/1
  robot_3_pose/1 -> Demux3/1
  Demux1/1 -> Scope1/1, MATLAB Function/1(x1)
  Demux1/2 -> MATLAB Function/2(y1), Scope1/2
  Demux/1 -> Scope2/1, MATLAB Function/3(z1)
  Demux2/1 -> MATLAB Function/4(x2)
  Demux2/2 -> MATLAB Function/5(y2)
  Demux/2 -> Scope2/2, MATLAB Function/6(z2)
  Demux3/1 -> MATLAB Function/7(x3)
  Demux3/2 -> MATLAB Function/8(y3)
  Demux/3 -> MATLAB Function/9(z3)
  MATLAB Function/1(x) -> Scope/1, x_velocity/1, Vector Concatenate/1
  MATLAB Function/2(y) -> Scope/2, y_velocity/1, Vector Concatenate/2

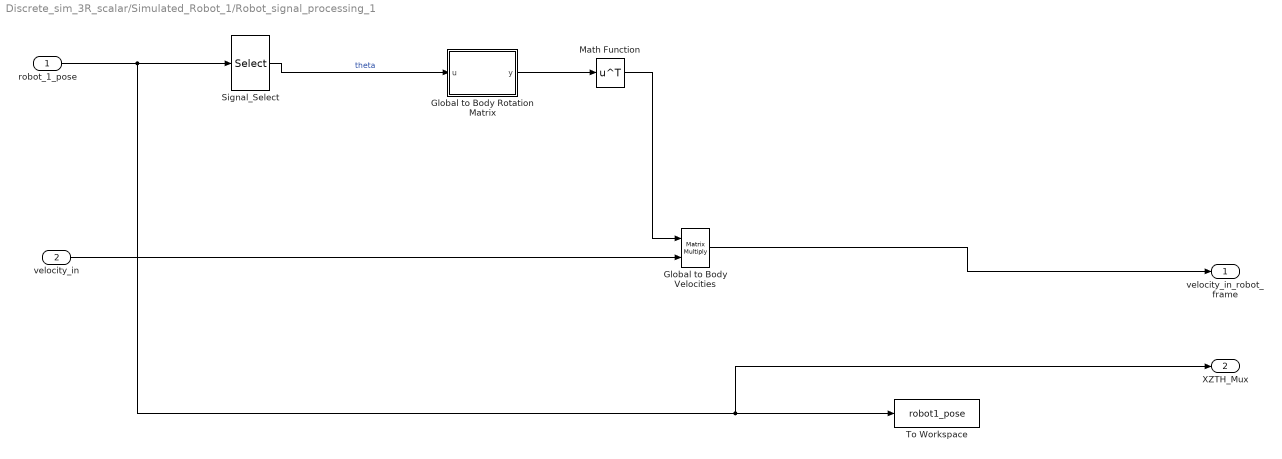
== system Discrete_sim_3R_scalar/Simulated_Robot_1/Robot_signal_processing_1 ==
  robot_1_pose : Inport
  velocity_in : Inport  Port=2
  Global to Body Velocities : Product  Multiplication=Matrix(*)
  Global to Body Rotation Matrix : MATLAB Function  TreatAsAtomicUnit=on
  Math Function : Math  Operator=transpose  SignedPower=on
  Signal_Select : Selector  InputPortWidth=3  IndexOptions=Index vector (dialog)  Indices=[3]  OutputSizes=1
  To Workspace : ToWorkspace  VariableName=robot1_pose  SaveFormat=Timeseries  SampleTime=-1
  velocity_in_robot_frame : Outport
  XZTH_Mux : Outport  Port=2
  wires:
  Signal_Select/1 -> Global to Body Rotation Matrix/1(u)  "theta"
  Global to Body Velocities/1 -> velocity_in_robot_frame/1
  robot_1_pose/1 -> XZTH_Mux/1, To Workspace/1, Signal_Select/1
  velocity_in/1 -> Global to Body Velocities/2
  Global to Body Rotation Matrix/1(y) -> Math Function/1
  Math Function/1 -> Global to Body Velocities/1

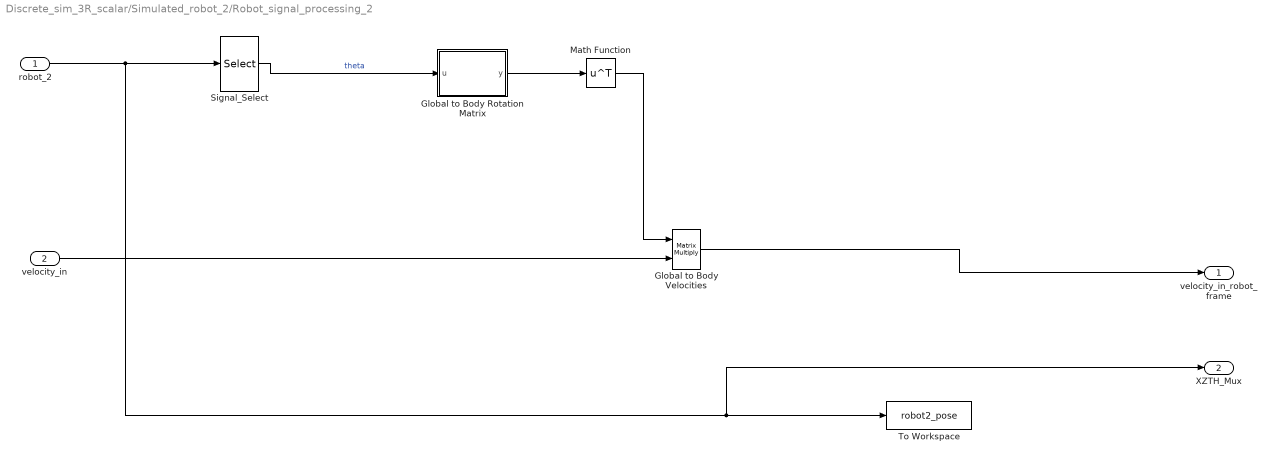
== system Discrete_sim_3R_scalar/Simulated_robot_2/Robot_signal_processing_2 ==
  robot_2 : Inport
  velocity_in : Inport  Port=2
  Global to Body Velocities : Product  Multiplication=Matrix(*)
  Global to Body Rotation Matrix : MATLAB Function  TreatAsAtomicUnit=on
  Math Function : Math  Operator=transpose  SignedPower=on
  Signal_Select : Selector  InputPortWidth=3  IndexOptions=Index vector (dialog)  Indices=[3]  OutputSizes=1
  To Workspace : ToWorkspace  VariableName=robot2_pose  SaveFormat=Timeseries  SampleTime=-1
  velocity_in_robot_frame : Outport
  XZTH_Mux : Outport  Port=2
  wires:
  Signal_Select/1 -> Global to Body Rotation Matrix/1(u)  "theta"
  Global to Body Velocities/1 -> velocity_in_robot_frame/1
  robot_2/1 -> XZTH_Mux/1, To Workspace/1, Signal_Select/1
  velocity_in/1 -> Global to Body Velocities/2
  Global to Body Rotation Matrix/1(y) -> Math Function/1
  Math Function/1 -> Global to Body Velocities/1

== system Discrete_sim_3R_scalar/Cluster_Controller_setpoint/P_Controller_or _control_Primitive/continous angle wrapping ==
  In1 : Inport
  Constant : Constant  Value=pi
  Constant1 : Constant  Value=2*pi
  Math Function : Math  Operator=mod  SignedPower=on
  Sum6 : Sum
  Sum7 : Sum  Inputs=-+
  Out1 : Outport
  wires:
  In1/1 -> Sum6/2
  Math Function/1 -> Sum7/2
  Constant/1 -> Sum7/1, Sum6/1
  Sum6/1 -> Math Function/1
  Constant1/1 -> Math Function/2
  Sum7/1 -> Out1/1

== matlab function Discrete_sim_3R_scalar/Cluster_Controller_countour/Cartesian to Cluster Variables ==
  data: fwdkin output; x1 input; x_c output; y1 input; th1 input; x2 input; y2 input; th2 input; x3 input; y3 input; th3 input; y_c output; th_c output; a output; b output; c output; phi1 output; phi2 output; phi3 output
function [fwdkin, x_c, y_c, th_c, a, b, c,phi1,phi2,phi3]   = Forward_Kinematics(x1, y1, th1, x2,y2,th2, x3,y3,th3)
% Centre frame
x_c = (x1+x2+x3)/3;
y_c = (y1+y2+y3)/3;
theta_c = atan2((2/3)*x1 - (1/3)*(x2 + x3), (2/3)*y1 - (1/3)*(y2 + y3));
% SAS Properties of triangle
p = sqrt((x1 - x2)^2 + (y1 - y2)^2);
q = sqrt((x3 - x1)^2 + (y1 - y3)^2);
beta = acos(((p^2 + q^2 - (x3 - x2)^2 - (y3 - y2)^2) / (2*p*q)));
% Rotation vectors
phi1 = th1 + theta_c;
phi2 = th2 + theta_c;
phi3 = th3 + theta_c;
a =p;
b = q;
c = beta;
th_c = theta_c;
fwdkin = [0 0 0 0 0 0];
fwdkin(1) =a;
fwdkin(2) =b;
fwdkin(3) =c;
fwdkin(4) =x_c;
fwdkin(5) =y_c;
fwdkin(6) =th_c;

== matlab function Discrete_sim_3R_scalar/Cluster_Controller_countour/Cluster Velocities to Cartesian Velocities ==
  data: fwdkin input; xc_err input; x1 output; zc_err input; thC_err input; a_err input; b_err input; C_err input; z1 output; th1 output; x2 output; z2 output; th2 output; x3 output; z3 output; th3 output
function [x1, z1,th1, x2,z2,th2, x3,z3, th3] = InverseJabobian(fwdkin, xc_err, zc_err, thC_err, a_err, b_err, C_err)
%% Unpacking the information from fwd_kin
p = fwdkin(1);
q = fwdkin(2);
beta = fwdkin(3);
xc = fwdkin(4);
yc = fwdkin(5);
theta_c = fwdkin(6);
yc_err = zc_err;
theta_c_err = thC_err;
p_err = a_err;
q_err = b_err;
beta_err = C_err;
%% Inverse Kinematics
  % Calculate x1, y1, and theta1 (Equations 12, 13, and 14)
r = sqrt((q + p*cos(beta))^2 + (p*sin(beta))^2);
  
x1 = xc + (1/3)*r*sin(theta_c);
y1 = yc + (1/3)*r*cos(theta_c);
%theta1 = phi1 - theta_c;
% Calculate x2, y2, and theta2 (Equations 15, 16, and 17)
x2 = xc + (1/3)*r*sin(theta_c) - p*sin(beta/2 + theta_c);
y2 = yc + (1/3)*r*cos(theta_c) - p*cos(beta/2 + theta_c);
%theta2 = phi2 - theta_c;
% Calculate x3, y3, and theta3 (Equations 18, 19, and 20)
x3 = xc + (1/3)*r*sin(theta_c) + q*sin(beta/2 - theta_c);
y3 = yc + (1/3)*r*cos(theta_c) - q*cos(beta/2 - theta_c);
%theta3 = phi3 - theta_c;
%% Now to take the partial derivates
% syms p q beta xc yc theta_c p_err q_err beta_err xc_err yc_err theta_c_err
% 
% % Define the equations
% eqs = [
%   xc + (1/3)*(sqrt((q + p*cos(beta))^2 + (p*sin(beta))^2))*sin(theta_c); % x1
%   yc + (1/3)*(sqrt((q + p*cos(beta))^2 + (p*sin(beta))^2))*cos(theta_c); % y1
%   xc + (1/3)*(sqrt((q + p*cos(beta))^2 + (p*sin(beta))^2))*sin(theta_c) - p*sin(beta/2 + theta_c); % x2
%   yc + (1/3)*(sqrt((q + p*cos(beta))^2 + (p*sin(beta))^2))*cos(theta_c) - p*cos(beta/2 + theta_c); % y2
%   xc + (1/3)*(sqrt((q + p*cos(beta))^2 + (p*sin(beta))^2))*sin(theta_c) + q*sin(beta/2 - theta_c); % x3
%   yc + (1/3)*(sqrt((q + p*cos(beta))^2 + (p*sin(beta))^2))*cos(theta_c) - q*cos(beta/2 - theta_c)  % y3
% ];
% 
% % Define the variables for differentiation
% vars = [p, q, beta, xc, yc, theta_c];
% 
% % Define the errors
% errs = [p_err, q_err, beta_err, xc_err, yc_err, theta_c_err];
% 
% % Initialize an array to store the sums (as symbolic)
% sums = sym(zeros(length(eqs), 1));
% 
% % Loop through equations and variables
% for i = 1:length(eqs)
%   for j = 1:length(vars)
%     derivative = diff(eqs(i), vars(j));
%     sums(i) = sums(i) + derivative * errs(j);
%   end
% end
% 
% % Display the results
% disp(simplify(sums(1)))
% disp(simplify(sums(2)))
% disp(simplify(sums(3)))
% disp(simplify(sums(4)))
% disp(simplify(sums(5)))
% disp(simplify(sums(6)))
%% Now to sum it all up
x1 =(3*xc_err*(p^2 + 2*cos(beta)*p*q + q^2)^(1/2) + p*p_err*sin(theta_c) + q*q_err*sin(theta_c) + p^2*theta_c_err*cos(theta_c) + q^2*theta_c_err*cos(theta_c) + p*q_err*cos(beta)*sin(theta_c) + p_err*q*cos(beta)*sin(theta_c) + 2*p*q*theta_c_err*cos(beta)*cos(theta_c) - beta_err*p*q*sin(beta)*sin(theta_c))/(3*(p^2 + 2*cos(beta)*p*q + q^2)^(1/2));
 
z1 = (3*yc_err*(p^2 + 2*cos(beta)*p*q + q^2)^(1/2) + p*p_err*cos(theta_c) + q*q_err*cos(theta_c) - p^2*theta_c_err*sin(theta_c) - q^2*theta_c_err*sin(theta_c) + p*q_err*cos(beta)*cos(theta_c) + p_err*q*cos(beta)*cos(theta_c) - beta_err*p*q*sin(beta)*cos(theta_c) - 2*p*q*theta_c_err*cos(beta)*sin(theta_c))/(3*(p^2 + 2*cos(beta)*p*q + q^2)^(1/2));
 
x2 = xc_err - p_err*(sin(beta/2 + theta_c) - (sin(theta_c)*(p + q*cos(beta)))/(3*(p^2 + 2*cos(beta)*p*q + q^2)^(1/2))) - beta_err*((p*cos(beta/2 + theta_c))/2 + (p*q*sin(beta)*sin(theta_c))/(3*(p^2 + 2*cos(beta)*p*q + q^2)^(1/2))) + theta_c_err*((cos(theta_c)*(p^2 + 2*cos(beta)*p*q + q^2)^(1/2))/3 - p*cos(beta/2 + theta_c)) + (q_err*sin(theta_c)*(q + p*cos(beta)))/(3*(p^2 + 2*cos(beta)*p*q + q^2)^(1/2));
 
z2 = yc_err - p_err*(cos(beta/2 + theta_c) - (cos(theta_c)*(p + q*cos(beta)))/(3*(p^2 + 2*cos(beta)*p*q + q^2)^(1/2))) + beta_err*((p*sin(beta/2 + theta_c))/2 - (p*q*sin(beta)*cos(theta_c))/(3*(p^2 + 2*cos(beta)*p*q + q^2)^(1/2))) - (theta_c_err*sin(theta_c)*(p^2 + 2*cos(beta)*p*q + q^2)^(1/2))/3 + p*theta_c_err*sin(beta/2 + theta_c) + (q_err*cos(theta_c)*(q + p*cos(beta)))/(3*(p^2 + 2*cos(beta)*p*q + q^2)^(1/2));
 
x3 = xc_err + q_err*(sin(beta/2 - theta_c) + (sin(theta_c)*(q + p*cos(beta)))/(3*(p^2 + 2*cos(beta)*p*q + q^2)^(1/2))) + beta_err*((q*cos(beta/2 - theta_c))/2 - (p*q*sin(beta)*sin(theta_c))/(3*(p^2 + 2*cos(beta)*p*q + q^2)^(1/2))) + (theta_c_err*cos(theta_c)*(p^2 + 2*cos(beta)*p*q + q^2)^(1/2))/3 - q*theta_c_err*cos(beta/2 - theta_c) + (p_err*sin(theta_c)*(p + q*cos(beta)))/(3*(p^2 + 2*cos(beta)*p*q + q^2)^(1/2));
 
z3 = yc_err - theta_c_err*(q*sin(beta/2 - theta_c) + (sin(theta_c)*(p^2 + 2*cos(beta)*p*q + q^2)^(1/2))/3) - q_err*(cos(beta/2 - theta_c) - (cos(theta_c)*(q + p*cos(beta)))/(3*(p^2 + 2*cos(beta)*p*q + q^2)^(1/2))) + beta_err*((q*sin(beta/2 - theta_c))/2 - (p*q*sin(beta)*cos(theta_c))/(3*(p^2 + 2*cos(beta)*p*q + q^2)^(1/2))) + (p_err*cos(theta_c)*(p + q*cos(beta)))/(3*(p^2 + 2*cos(beta)*p*q + q^2)^(1/2));
 
th1 = 0;
th2 = 0;
th3 = 0;

== matlab function Discrete_sim_3R_scalar/Robot1_Sensor_output to height/Mountain ==
  data: sensor_output input; height output
function height = simulated_readings(sensor_output)

height = (sensor_output+ 0.3)*1.5;

end

== matlab function Discrete_sim_3R_scalar/Simulated_robot_2/Same Crater ==
  data: x input; sensor_output output; z input; th input
function sensor_output = simulated__environmental_readings(x,z,th)

sensor_output= (((x^2 + z^2)^0.5)*.54) + 0.3;

end

== matlab function Discrete_sim_3R_scalar/Robot1_Sensor_output to height1/Mountain ==
  data: sensor_output input; height output
function height = simulated_readings(sensor_output)

height = (sensor_output+ 0.3)*1.5;

end

== matlab function Discrete_sim_3R_scalar/model of the environment and robot 3 reading from it ==
  data: x input; sensor_output output; z input; th input
function sensor_output = simulated__environmental_readings(x,z,th)

sensor_output= (((x^2 + z^2)^0.5)*.54) + 0.3;

end

== matlab function Discrete_sim_3R_scalar/Robot1_Sensor_output to height2/Mountain ==
  data: sensor_output input; height output
function height = simulated_readings(sensor_output)

height = (sensor_output+ 0.3)*1.5;

end

== matlab function Discrete_sim_3R_scalar/Estimator for robot 1 (In this case, a perfect estimator)/Same Crater Yet Again ==
  data: x input; sensor_output output; z input; th input
function sensor_output = simulated__environmental_readings(x,z,th)

sensor_output= (((x^2 + z^2)^0.5)*.54) + 0.3;

end

== matlab function Discrete_sim_3R_scalar/Cluster_Controller_countour/contour_following/MATLAB Function ==
  data: x output; x1 input; y output; y1 input; z1 input; x2 input; y2 input; z2 input; x3 input; y3 input; z3 input
function [x, y] = countourfollowing(x1, y1, z1, x2, y2, z2, x3, y3, z3)
  % Create vectors AB and AC
  AB = [x2 - x1, y2 - y1, z2 - z1];
  AC = [x3 - x1, y3 - y1, z3 - z1];

  % Calculate the cross product to get the normal vector
  N = cross(-AB, AC);

  % Get the direction of steepest descent (-N)
  descent =-N ;

  % Normalize the vector to have unit length in the xy-plane
  magnitude = sqrt(descent(1)^2 + descent(2)^2);
  x = descent(1) / magnitude;
  y = descent(2) / magnitude;

  x = x*.5;
  y = y*.5;


  %% Rotation by 90 degrees
  x1 = x;
  y1 = y;

  y = x1;
  x = -y1;

end

== matlab function Discrete_sim_3R_scalar/Cluster_Controller_steepest_descent/gradient_ascent/MATLAB Function ==
  data: x output; x1 input; y output; y1 input; z1 input; x2 input; y2 input; z2 input; x3 input; y3 input; z3 input
function [x, y] = steepestDescent(x1, y1, z1, x2, y2, z2, x3, y3, z3)
  % Create vectors AB and AC
  AB = [x2 - x1, y2 - y1, z2 - z1];
  AC = [x3 - x1, y3 - y1, z3 - z1];

  % Calculate the cross product to get the normal vector
  N = cross(-AB, AC);

  % Get the direction of steepest descent (-N)
  descent =-N;

  % Normalize the vector to have unit length in the xy-plane
  magnitude = sqrt(descent(1)^2 + descent(2)^2);
  x = descent(1) / magnitude;
  y = descent(2) / magnitude;
  x = x/10;
  y = y/10;
end

== matlab function Discrete_sim_3R_scalar/Cluster_Controller_steepest_descent/Cartesian to Cluster Variables ==
  data: fwdkin output; x1 input; x_c output; y1 input; th1 input; x2 input; y2 input; th2 input; x3 input; y3 input; th3 input; y_c output; th_c output; a output; b output; c output; phi1 output; phi2 output; phi3 output
function [fwdkin, x_c, y_c, th_c, a, b, c,phi1,phi2,phi3]   = Forward_Kinematics(x1, y1, th1, x2,y2,th2, x3,y3,th3)
% Centre frame
x_c = (x1+x2+x3)/3;
y_c = (y1+y2+y3)/3;
theta_c = atan2((2/3)*x1 - (1/3)*(x2 + x3), (2/3)*y1 - (1/3)*(y2 + y3));
% SAS Properties of triangle
p = sqrt((x1 - x2)^2 + (y1 - y2)^2);
q = sqrt((x3 - x1)^2 + (y1 - y3)^2);
beta = acos((p^2 + q^2 - (x3 - x2)^2 - (y3 - y2)^2) / (2*p*q));
% Rotation vectors
phi1 = th1 + theta_c;
phi2 = th2 + theta_c;
phi3 = th3 + theta_c;
a =p;
b = q;
c = beta;
th_c = theta_c;
fwdkin = [0 0 0 0 0 0];
fwdkin(1) =a;
fwdkin(2) =b;
fwdkin(3) =c;
fwdkin(4) =x_c;
fwdkin(5) =y_c;
fwdkin(6) =th_c;

== matlab function Discrete_sim_3R_scalar/Simulated_Robot_1/Crater ==
  data: x input; sensor_output output; z input; th input
function sensor_output = simulated__environmental_readings(x,z,th)

sensor_output= (((x^2 + z^2)^0.5)*.54) + 0.3;

end

== matlab function Discrete_sim_3R_scalar/Simulated_robot_2/Robot_signal_processing_2/Global to Body Rotation Matrix ==
  data: u input; y output
function y = fcn(u)

y = [cos(u) -sin(u) 0; sin(u) cos(u) 0; 0 0 1];

== matlab function Discrete_sim_3R_scalar/Robot_3_Dynamics/Global to Body Rotation Matrix ==
  data: u input; y output
function y = fcn(u)

y = [cos(u) -sin(u) 0; sin(u) cos(u) 0; 0 0 1];

== matlab function Discrete_sim_3R_scalar/Cluster_Controller_setpoint/Cartesian to Cluster Variables ==
  data: fwdkin output; x1 input; x_c output; y1 input; th1 input; x2 input; y2 input; th2 input; x3 input; y3 input; th3 input; y_c output; th_c output; a output; b output; c output
function [fwdkin, x_c, y_c, th_c, a, b, c]   = Forward_Kinematics(x1, y1, th1, x2,y2,th2, x3,y3,th3)
% Centre frame
x_c = (x1+x2+x3)/3;
y_c = (y1+y2+y3)/3;
theta_c = atan2((2/3)*x1 - (1/3)*(x2 + x3), (2/3)*y1 - (1/3)*(y2 + y3));
% SAS Properties of triangle
p = sqrt((x1 - x2)^2 + (y1 - y2)^2);
q = sqrt((x3 - x1)^2 + (y1 - y3)^2);
beta = acos((p^2 + q^2 - (x3 - x2)^2 - (y3 - y2)^2) / (2*p*q));
% Rotation vectors
phi1 = th1 + theta_c;
phi2 = th2 + theta_c;
phi3 = th3 + theta_c;
a =p;
b = q;
c = beta;
th_c = theta_c;
fwdkin = [0 0 0 0 0 0];
fwdkin(1) =a;
fwdkin(2) =b;
fwdkin(3) =c;
fwdkin(4) =x_c;
fwdkin(5) =y_c;
fwdkin(6) =th_c;

== matlab function Discrete_sim_3R_scalar/Cluster_Controller_setpoint/Cluster Velocities to Cartesian Velocities ==
  data: fwdkin input; xc_err input; x1 output; zc_err input; thC_err input; a_err input; b_err input; C_err input; z1 output; th1 output; x2 output; z2 output; th2 output; x3 output; z3 output; th3 output
function [x1, z1,th1, x2,z2,th2, x3,z3, th3] = InverseJabobian(fwdkin, xc_err, zc_err, thC_err, a_err, b_err, C_err)
%% Unpacking the information from fwd_kin
p = fwdkin(1);
q = fwdkin(2);
beta = fwdkin(3);
xc = fwdkin(4);
yc = fwdkin(5);
theta_c = fwdkin(6);
yc_err = zc_err;
theta_c_err = thC_err;
p_err = a_err;
q_err = b_err;
beta_err = C_err;
%% Inverse Kinematics
  % Calculate x1, y1, and theta1 (Equations 12, 13, and 14)
r = sqrt((q + p*cos(beta))^2 + (p*sin(beta))^2);
  
x1 = xc + (1/3)*r*sin(theta_c);
y1 = yc + (1/3)*r*cos(theta_c);
%theta1 = phi1 - theta_c;
% Calculate x2, y2, and theta2 (Equations 15, 16, and 17)
x2 = xc + (1/3)*r*sin(theta_c) - p*sin(beta/2 + theta_c);
y2 = yc + (1/3)*r*cos(theta_c) - p*cos(beta/2 + theta_c);
%theta2 = phi2 - theta_c;
% Calculate x3, y3, and theta3 (Equations 18, 19, and 20)
x3 = xc + (1/3)*r*sin(theta_c) + q*sin(beta/2 - theta_c);
y3 = yc + (1/3)*r*cos(theta_c) - q*cos(beta/2 - theta_c);
%theta3 = phi3 - theta_c;
%% Now to take the partial derivates
% syms p q beta xc yc theta_c p_err q_err beta_err xc_err yc_err theta_c_err
% 
% % Define the equations
% eqs = [
%   xc + (1/3)*(sqrt((q + p*cos(beta))^2 + (p*sin(beta))^2))*sin(theta_c); % x1
%   yc + (1/3)*(sqrt((q + p*cos(beta))^2 + (p*sin(beta))^2))*cos(theta_c); % y1
%   xc + (1/3)*(sqrt((q + p*cos(beta))^2 + (p*sin(beta))^2))*sin(theta_c) - p*sin(beta/2 + theta_c); % x2
%   yc + (1/3)*(sqrt((q + p*cos(beta))^2 + (p*sin(beta))^2))*cos(theta_c) - p*cos(beta/2 + theta_c); % y2
%   xc + (1/3)*(sqrt((q + p*cos(beta))^2 + (p*sin(beta))^2))*sin(theta_c) + q*sin(beta/2 - theta_c); % x3
%   yc + (1/3)*(sqrt((q + p*cos(beta))^2 + (p*sin(beta))^2))*cos(theta_c) - q*cos(beta/2 - theta_c)  % y3
% ];
% 
% % Define the variables for differentiation
% vars = [p, q, beta, xc, yc, theta_c];
% 
% % Define the errors
% errs = [p_err, q_err, beta_err, xc_err, yc_err, theta_c_err];
% 
% % Initialize an array to store the sums (as symbolic)
% sums = sym(zeros(length(eqs), 1));
% 
% % Loop through equations and variables
% for i = 1:length(eqs)
%   for j = 1:length(vars)
%     derivative = diff(eqs(i), vars(j));
%     sums(i) = sums(i) + derivative * errs(j);
%   end
% end
% 
% % Display the results
% disp(simplify(sums(1)))
% disp(simplify(sums(2)))
% disp(simplify(sums(3)))
% disp(simplify(sums(4)))
% disp(simplify(sums(5)))
% disp(simplify(sums(6)))
%% Now to sum it all up
x1 =(3*xc_err*(p^2 + 2*cos(beta)*p*q + q^2)^(1/2) + p*p_err*sin(theta_c) + q*q_err*sin(theta_c) + p^2*theta_c_err*cos(theta_c) + q^2*theta_c_err*cos(theta_c) + p*q_err*cos(beta)*sin(theta_c) + p_err*q*cos(beta)*sin(theta_c) + 2*p*q*theta_c_err*cos(beta)*cos(theta_c) - beta_err*p*q*sin(beta)*sin(theta_c))/(3*(p^2 + 2*cos(beta)*p*q + q^2)^(1/2));
 
z1 = (3*yc_err*(p^2 + 2*cos(beta)*p*q + q^2)^(1/2) + p*p_err*cos(theta_c) + q*q_err*cos(theta_c) - p^2*theta_c_err*sin(theta_c) - q^2*theta_c_err*sin(theta_c) + p*q_err*cos(beta)*cos(theta_c) + p_err*q*cos(beta)*cos(theta_c) - beta_err*p*q*sin(beta)*cos(theta_c) - 2*p*q*theta_c_err*cos(beta)*sin(theta_c))/(3*(p^2 + 2*cos(beta)*p*q + q^2)^(1/2));
 
x2 = xc_err - p_err*(sin(beta/2 + theta_c) - (sin(theta_c)*(p + q*cos(beta)))/(3*(p^2 + 2*cos(beta)*p*q + q^2)^(1/2))) - beta_err*((p*cos(beta/2 + theta_c))/2 + (p*q*sin(beta)*sin(theta_c))/(3*(p^2 + 2*cos(beta)*p*q + q^2)^(1/2))) + theta_c_err*((cos(theta_c)*(p^2 + 2*cos(beta)*p*q + q^2)^(1/2))/3 - p*cos(beta/2 + theta_c)) + (q_err*sin(theta_c)*(q + p*cos(beta)))/(3*(p^2 + 2*cos(beta)*p*q + q^2)^(1/2));
 
z2 = yc_err - p_err*(cos(beta/2 + theta_c) - (cos(theta_c)*(p + q*cos(beta)))/(3*(p^2 + 2*cos(beta)*p*q + q^2)^(1/2))) + beta_err*((p*sin(beta/2 + theta_c))/2 - (p*q*sin(beta)*cos(theta_c))/(3*(p^2 + 2*cos(beta)*p*q + q^2)^(1/2))) - (theta_c_err*sin(theta_c)*(p^2 + 2*cos(beta)*p*q + q^2)^(1/2))/3 + p*theta_c_err*sin(beta/2 + theta_c) + (q_err*cos(theta_c)*(q + p*cos(beta)))/(3*(p^2 + 2*cos(beta)*p*q + q^2)^(1/2));
 
x3 = xc_err + q_err*(sin(beta/2 - theta_c) + (sin(theta_c)*(q + p*cos(beta)))/(3*(p^2 + 2*cos(beta)*p*q + q^2)^(1/2))) + beta_err*((q*cos(beta/2 - theta_c))/2 - (p*q*sin(beta)*sin(theta_c))/(3*(p^2 + 2*cos(beta)*p*q + q^2)^(1/2))) + (theta_c_err*cos(theta_c)*(p^2 + 2*cos(beta)*p*q + q^2)^(1/2))/3 - q*theta_c_err*cos(beta/2 - theta_c) + (p_err*sin(theta_c)*(p + q*cos(beta)))/(3*(p^2 + 2*cos(beta)*p*q + q^2)^(1/2));
 
z3 = yc_err - theta_c_err*(q*sin(beta/2 - theta_c) + (sin(theta_c)*(p^2 + 2*cos(beta)*p*q + q^2)^(1/2))/3) - q_err*(cos(beta/2 - theta_c) - (cos(theta_c)*(q + p*cos(beta)))/(3*(p^2 + 2*cos(beta)*p*q + q^2)^(1/2))) + beta_err*((q*sin(beta/2 - theta_c))/2 - (p*q*sin(beta)*cos(theta_c))/(3*(p^2 + 2*cos(beta)*p*q + q^2)^(1/2))) + (p_err*cos(theta_c)*(p + q*cos(beta)))/(3*(p^2 + 2*cos(beta)*p*q + q^2)^(1/2));
 
th1 = 0;
th2 = 0;
th3 = 0;

== matlab function Discrete_sim_3R_scalar/Simulated_Robot_1/Robot_signal_processing_1/Global to Body Rotation Matrix ==
  data: u input; y output
function y = fcn(u)

y = [cos(u) -sin(u) 0; sin(u) cos(u) 0; 0 0 1];
